simulink model "IEEE34bus_2subsystem"  (R2022b)
settings: Solver=ode4  StartTime=0.0  StopTime=inf  FixedStep=Ts  MaxStep=1e-4  RelTol=1e-4
InitFcn:
  | a=1; % Loading Factor
  | Ts=50e-6;
  | % phase to sequence conversion of RXB matrices
  | c=1*exp(sqrt(-1)*(120*pi/180));
  | T=[1 1 1;1 c*c c;1 c c*c];
  | Tinv=1/3*[1 1 1;1 c c*c;1 c*c c];
  | 
  | % Simulation data for the IEEE 34 Node Test Feeder model
  | mi2km = 1.60934;%  miles to km conversion
  | ft2km = 0.0003048; % feet to km conversion
  | ms2F = 1*1e-6/(2*pi*60);% microsiemens to Farads conversion
  | 
  | %% Configuration 300 - series reactance - ohm/mile
  | R_300 = [1.3368 0.2101 0.2130;0.2101 1.3238 0.2066;0.2130 0.2066 1.3294];
  | X_300 = [1.3343 0.5779 0.5015;0.5779 1.3569 0.4591;0.5015 0.4591 1.3471];
  | % charging susceptance - microsiemens/mile
  | B_300 = [5.3350 -1.5313 -0.9943;-1.5313 5.0979 -0.6212;-0.9943 -0.6212 4.8880];
  | 
  | R_300 = R_300/mi2km;
  | Rseq=Tinv*R_300*T;
  | R1_300=Rseq(2,2);R0_300=Rseq(1,1);
  | 
  | L_300 = (X_300/(2*pi*60))/mi2km;
  | Lseq=Tinv*L_300*T;
  | L1_300=Lseq(2,2);L0_300=Lseq(1,1);
  | 
  | C_300 =(B_300*ms2F)/mi2km;
  | Cseq=Tinv*C_300*T;
  | C1_300=Cseq(2,2);C0_300=Cseq(1,1);
  | 
  | %% Configuration 301 - series reactance - ohm/mile
  | R_301 = [1.9300 0.2327 0.2359;0.2327 1.9157 0.2288;0.2359 0.2288 1.9219];
  | X_301 = [1.4115 0.6442 0.5691;0.6442 1.4281 0.5238;0.5691 0.5238 1.4209];
  | % charging susceptance - microsiemens/mile
  | B_301 = [5.1207 -1.4364 -0.9402;-1.4364 4.9055 -0.5951;-0.9402 -0.5951 4.7154];
  | 
  | R_301 = R_301/mi2km;
  | Rseq=Tinv*R_301*T;
  | R1_301=Rseq(2,2);R0_301=Rseq(1,1);
  | 
  | L_301 = (X_301/(2*pi*60))/mi2km;
  | Lseq=Tinv*L_301*T;
  | L1_301=Lseq(2,2);L0_301=Lseq(1,1);
  | 
  | C_301 =(B_301*ms2F)/mi2km;
  | Cseq=Tinv*C_301*T;
  | C1_301=Cseq(2,2);C0_301=Cseq(1,1);
  | 
  | %% Configuration 302 - series reactance - ohm/mile
  | R_302 = [2.7995 0 0;0 0 0;0 0 0];
  | X_302 = [1.4855 0 0;0 0 0;0 0 0];
  | % charging susceptance - microsiemens/mile
  | B_302 = [4.2251 0 0;0 0 0;0 0 0];
  | 
  | R_302 = R_302/mi2km;
  | Rseq=Tinv*R_302*T;
  | R1_302=Rseq(2,2);R0_302=Rseq(1,1);
  | 
  | L_302 = (X_302/(2*pi*60))/mi2km;
  | Lseq=Tinv*L_302*T;
  | ... (+41 lines)
undefined symbols (not defined in the file): find_system, I, Left, MOV_segment19, MOV_segment9, powergui, Right, type, V, X, xn_g1
libraries: spsSeriesRLCBranchLib x75, spsGroundLib x70, spsThreePhaseVIMeasurementLib x37, spsVoltageMeasurementLib x36, spsThreePhaseSeriesRLCLoadLib x32, spsThreePhasePISectionLineLib x24, spsDCVoltageSourceLib x24, ssn_lib x16, spsSeriesRLCLoadLib x14, spsACCurrentSourceLib x12, spsOnDelayLib x12, spsPiSectionLineLib x8
(part 3 of 8)

== system IEEE34bus_2subsystem/SS_34p1/838 ==
  1 : spsThreePhaseVIMeasurementLib/Three-Phase V-I Measurement  VoltageMeasurement=phase-to-ground  SetLabelV=on  LabelV=V838  Vpu=off  VpuLL=off  CurrentMeasurement=no  SetLabelI=on  LabelI=I862  Ipu=off  Pbase=100e6  Vbase=24900  OutputType=Complex  PhasorSimulation=off  PSBequivalent=0
  Ground{1..2,9,12} (4 alike) : spsGroundLib/Ground  LConnTagsString=a
  b : PMIOPort  Side=Left
  B : PMIOPort  Port=2  Side=Right
  connections:
  1/LConn2 -- B/RConn1
  Ground12/LConn1 -- 1/LConn1
  b/RConn1 -- 1/RConn2
  Ground9/LConn1 -- 1/RConn1
  Ground2/LConn1 -- 1/LConn3
  Ground1/LConn1 -- 1/RConn3

== system IEEE34bus_2subsystem/powergui/EquivalentModel1 ==
  Sources : Subsystem
  State-Space : S-Function  FunctionName=ssn_sfun_v1  Parameters=1,0  SFunctionDeploymentMode=off  EnableBusSupport=off  SFcnStateName=MOV_segment9,MOV_segment9,MOV_segment9,MOV_segment9,MOV_segment9,MOV_segment9,MOV_segment9,MOV_segment9,MOV_segment9,MOV_segment9
      settings: SFcnIsStateOwnerBlock=on
  Yout : Subsystem
  wires:
  State-Space/1 -> Yout/1(v,i)
  Sources/1(u) -> State-Space/1

== system IEEE34bus_2subsystem/powergui/EquivalentModel2 ==
  Sources : Subsystem
  State-Space : S-Function  FunctionName=ssn_sfun_v1  Parameters=2,0  SFunctionDeploymentMode=off  EnableBusSupport=off  SFcnStateName=MOV_segment9,MOV_segment9,MOV_segment9,MOV_segment9,MOV_segment9,MOV_segment9,MOV_segment9,MOV_segment9,MOV_segment9,MOV_segment9
      settings: SFcnIsStateOwnerBlock=on
  Yout : Subsystem
  wires:
  State-Space/1 -> Yout/1(v,i)
  Sources/1(u) -> State-Space/1

== system IEEE34bus_2subsystem/powergui/EquivalentModel3 ==
  Sources : Subsystem
  State-Space : S-Function  FunctionName=ssn_sfun_v1  Parameters=3,0  SFunctionDeploymentMode=off  EnableBusSupport=off  SFcnStateName=MOV_segment9,MOV_segment9,MOV_segment9,MOV_segment9,MOV_segment9,MOV_segment9,MOV_segment9,MOV_segment9,MOV_segment9,MOV_segment9
      settings: SFcnIsStateOwnerBlock=on
  Yout : Subsystem
  wires:
  State-Space/1 -> Yout/1(v,i)
  Sources/1(u) -> State-Space/1

== system IEEE34bus_2subsystem/powergui/EquivalentModel4 ==
  Sources : Subsystem
  State-Space : S-Function  FunctionName=ssn_sfun_v1  Parameters=4,0  SFunctionDeploymentMode=off  EnableBusSupport=off  SFcnStateName=MOV_segment9,MOV_segment9,MOV_segment9,MOV_segment9,MOV_segment9,MOV_segment9,MOV_segment9,MOV_segment9,MOV_segment9,MOV_segment9
      settings: SFcnIsStateOwnerBlock=on
  Yout : Subsystem
  wires:
  State-Space/1 -> Yout/1(v,i)
  Sources/1(u) -> State-Space/1

== system IEEE34bus_2subsystem/powergui/EquivalentModel5 ==
  Sources : Subsystem
  State-Space : S-Function  FunctionName=ssn_sfun_v1  Parameters=5,0  SFunctionDeploymentMode=off  EnableBusSupport=off  SFcnStateName=MOV_segment9,MOV_segment9,MOV_segment9,MOV_segment9,MOV_segment9,MOV_segment9,MOV_segment9,MOV_segment9,MOV_segment9,MOV_segment9
      settings: SFcnIsStateOwnerBlock=on
  Yout : Subsystem
  wires:
  State-Space/1 -> Yout/1(v,i)
  Sources/1(u) -> State-Space/1

== system IEEE34bus_2subsystem/powergui/EquivalentModel6 ==
  Sources : Subsystem
  State-Space : S-Function  FunctionName=ssn_sfun_v1  Parameters=6,0  SFunctionDeploymentMode=off  EnableBusSupport=off  SFcnStateName=MOV_segment9,MOV_segment9,MOV_segment9,MOV_segment9,MOV_segment9,MOV_segment9,MOV_segment9,MOV_segment9,MOV_segment9,MOV_segment9
      settings: SFcnIsStateOwnerBlock=on
  Yout : Subsystem
  wires:
  State-Space/1 -> Yout/1(v,i)
  Sources/1(u) -> State-Space/1

== system IEEE34bus_2subsystem/powergui/EquivalentModel7 ==
  Sources : Subsystem
  State-Space : Subsystem
  Yout : Subsystem
  wires:
  State-Space/1(Out1) -> Yout/1(v,i)
  Sources/1(u) -> State-Space/1(In1)

== system IEEE34bus_2subsystem/powergui/EquivalentModel8 ==
  Sources : Subsystem
  State-Space : S-Function  FunctionName=ssn_sfun_v1  Parameters=8,0  SFunctionDeploymentMode=off  EnableBusSupport=off  SFcnStateName=MOV_segment19,xn_g1,MOV_segment19,MOV_segment19,MOV_segment19,MOV_segment19,MOV_segment19,MOV_segment19,MOV_segment19,MOV_segment19,MOV_segment19,MOV_segment19,MOV_segment19,MOV_segment19,MOV_segment19,MOV_segment19,MOV_segment19,MOV_segment19,MOV_segment19,MOV_segment19
      settings: SFcnIsStateOwnerBlock=on
  Yout : Subsystem
  wires:
  State-Space/1 -> Yout/1(v,i)
  Sources/1(u) -> State-Space/1

== system IEEE34bus_2subsystem/SM_34p/Regulator 3/Single Phase SVR_A ==
  Line Drop Compensator : Subsystem
  Transformer with Taps : Subsystem
  Voltage Regulator Control : Subsystem
  S : PMIOPort  Tag=PMCPort  Side=Left
  L : PMIOPort  Tag=PMCPort  Port=2  Side=Right
  Tap : Outport  VectorParamsAs1DForOutWhenUnconnected=off
  tag scope: Vr1a=global
  wires:
  Transformer with Taps/2(Vsec) -> Line Drop Compensator/2(Vsec)
  Transformer with Taps/1(Isec) -> Line Drop Compensator/1(Isec)
  Voltage Regulator Control/1(N) -> Transformer with Taps/1(N)
  Voltage Regulator Control/2(Tap) -> Tap/1
  Line Drop Compensator/1(Vm) -> [Vr1a], Voltage Regulator Control/1(Vm)
  connections:
  Transformer with Taps/LConn1 -- S/RConn1
  Transformer with Taps/RConn1 -- L/RConn1

== system IEEE34bus_2subsystem/SM_34p/Regulator 3/Single Phase SVR_B ==
  Line Drop Compensator : Subsystem
  Transformer with Taps : Subsystem
  Voltage Regulator Control : Subsystem
  S : PMIOPort  Tag=PMCPort  Side=Left
  L : PMIOPort  Tag=PMCPort  Port=2  Side=Right
  Tap : Outport  VectorParamsAs1DForOutWhenUnconnected=off
  tag scope: Vr1b=global
  wires:
  Line Drop Compensator/1(Vm) -> Voltage Regulator Control/1(Vm), [Vr1b]
  Voltage Regulator Control/2(Tap) -> Tap/1
  Voltage Regulator Control/1(N) -> Transformer with Taps/1(N)
  Transformer with Taps/1(Isec) -> Line Drop Compensator/1(Isec)
  Transformer with Taps/2(Vsec) -> Line Drop Compensator/2(Vsec)
  connections:
  Transformer with Taps/RConn1 -- L/RConn1
  Transformer with Taps/LConn1 -- S/RConn1

== system IEEE34bus_2subsystem/SM_34p/Regulator 3/Single Phase SVR_C ==
  Line Drop Compensator : Subsystem
  Transformer with Taps : Subsystem
  Voltage Regulator Control : Subsystem
  S : PMIOPort  Tag=PMCPort  Side=Left
  L : PMIOPort  Tag=PMCPort  Port=2  Side=Right
  Tap : Outport  VectorParamsAs1DForOutWhenUnconnected=off
  tag scope: Vr1c=global
  wires:
  Transformer with Taps/2(Vsec) -> Line Drop Compensator/2(Vsec)
  Transformer with Taps/1(Isec) -> Line Drop Compensator/1(Isec)
  Voltage Regulator Control/1(N) -> Transformer with Taps/1(N)
  Voltage Regulator Control/2(Tap) -> Tap/1
  Line Drop Compensator/1(Vm) -> [Vr1c], Voltage Regulator Control/1(Vm)
  connections:
  Transformer with Taps/LConn1 -- S/RConn1
  Transformer with Taps/RConn1 -- L/RConn1

== system IEEE34bus_2subsystem/SM_34p/Regulator 4/Single Phase SVR_A ==
  Line Drop Compensator : Subsystem
  Transformer with Taps : Subsystem
  Voltage Regulator Control : Subsystem
  S : PMIOPort  Tag=PMCPort  Side=Left
  L : PMIOPort  Tag=PMCPort  Port=2  Side=Right
  Tap : Outport  VectorParamsAs1DForOutWhenUnconnected=off
  tag scope: Vr2a=global
  wires:
  Line Drop Compensator/1(Vm) -> Voltage Regulator Control/1(Vm), [Vr2a]
  Voltage Regulator Control/2(Tap) -> Tap/1
  Voltage Regulator Control/1(N) -> Transformer with Taps/1(N)
  Transformer with Taps/1(Isec) -> Line Drop Compensator/1(Isec)
  Transformer with Taps/2(Vsec) -> Line Drop Compensator/2(Vsec)
  connections:
  Transformer with Taps/RConn1 -- L/RConn1
  Transformer with Taps/LConn1 -- S/RConn1

== system IEEE34bus_2subsystem/SM_34p/Regulator 4/Single Phase SVR_B ==
  Line Drop Compensator : Subsystem
  Transformer with Taps : Subsystem
  Voltage Regulator Control : Subsystem
  S : PMIOPort  Tag=PMCPort  Side=Left
  L : PMIOPort  Tag=PMCPort  Port=2  Side=Right
  Tap : Outport  VectorParamsAs1DForOutWhenUnconnected=off
  tag scope: Vr2b=global
  wires:
  Transformer with Taps/2(Vsec) -> Line Drop Compensator/2(Vsec)
  Transformer with Taps/1(Isec) -> Line Drop Compensator/1(Isec)
  Voltage Regulator Control/1(N) -> Transformer with Taps/1(N)
  Voltage Regulator Control/2(Tap) -> Tap/1
  Line Drop Compensator/1(Vm) -> [Vr2b], Voltage Regulator Control/1(Vm)
  connections:
  Transformer with Taps/LConn1 -- S/RConn1
  Transformer with Taps/RConn1 -- L/RConn1

== system IEEE34bus_2subsystem/SM_34p/Regulator 4/Single Phase SVR_C ==
  Line Drop Compensator : Subsystem
  Transformer with Taps : Subsystem
  Voltage Regulator Control : Subsystem
  S : PMIOPort  Tag=PMCPort  Side=Left
  L : PMIOPort  Tag=PMCPort  Port=2  Side=Right
  Tap : Outport  VectorParamsAs1DForOutWhenUnconnected=off
  tag scope: Vr2c=global
  wires:
  Line Drop Compensator/1(Vm) -> Voltage Regulator Control/1(Vm), [Vr2c]
  Voltage Regulator Control/2(Tap) -> Tap/1
  Voltage Regulator Control/1(N) -> Transformer with Taps/1(N)
  Transformer with Taps/1(Isec) -> Line Drop Compensator/1(Isec)
  Transformer with Taps/2(Vsec) -> Line Drop Compensator/2(Vsec)
  connections:
  Transformer with Taps/RConn1 -- L/RConn1
  Transformer with Taps/LConn1 -- S/RConn1

== system IEEE34bus_2subsystem/powergui/EquivalentModel1/Sources ==
  Mux : Mux  Inputs=[1 1]
  u : Outport  VectorParamsAs1DForOutWhenUnconnected=off
  wires:
  Mux/1 -> u/1
  [T91_7975_12543828221255] -> Mux/1
  [T91_7962_12463308468462] -> Mux/2

== system IEEE34bus_2subsystem/powergui/EquivalentModel1/Yout ==
  v,i : Inport
  Demux : Demux  Outputs=1
  tag scope: T94_8507_15463232269065=global
  wires:
  v,i/1 -> Demux/1
  Demux/1 -> [T94_8507_15463232269065]

== system IEEE34bus_2subsystem/powergui/EquivalentModel2/Sources ==
  Mux : Mux  Inputs=[1 1]
  u : Outport  VectorParamsAs1DForOutWhenUnconnected=off
  wires:
  Mux/1 -> u/1
  [T91_7976_12543360980049] -> Mux/1
  [T91_7963_12462866570525] -> Mux/2

== system IEEE34bus_2subsystem/powergui/EquivalentModel2/Yout ==
  v,i : Inport
  Demux : Demux  Outputs=1
  tag scope: T94_8508_15461981939973=global
  wires:
  v,i/1 -> Demux/1
  Demux/1 -> [T94_8508_15461981939973]

== system IEEE34bus_2subsystem/powergui/EquivalentModel3/Sources ==
  Mux : Mux  Inputs=[1 1]
  u : Outport  VectorParamsAs1DForOutWhenUnconnected=off
  wires:
  Mux/1 -> u/1
  [T91_7977_12543017695106] -> Mux/1
  [T91_7964_12462548628852] -> Mux/2

== system IEEE34bus_2subsystem/powergui/EquivalentModel3/Yout ==
  v,i : Inport
  Demux : Demux  Outputs=1
  tag scope: T94_8509_15460851611092=global
  wires:
  v,i/1 -> Demux/1
  Demux/1 -> [T94_8509_15460851611092]

== system IEEE34bus_2subsystem/powergui/EquivalentModel4/Sources ==
  Mux : Mux  Inputs=[1 1]
  u : Outport  VectorParamsAs1DForOutWhenUnconnected=off
  wires:
  Mux/1 -> u/1
  [T91_7976_12540912541255] -> Mux/1
  [T91_7963_12460409796462] -> Mux/2

== system IEEE34bus_2subsystem/powergui/EquivalentModel4/Yout ==
  v,i : Inport
  Demux : Demux  Outputs=1
  tag scope: T94_8508_15459874989120=global
  wires:
  v,i/1 -> Demux/1
  Demux/1 -> [T94_8508_15459874989120]

== system IEEE34bus_2subsystem/powergui/EquivalentModel5/Sources ==
  Mux : Mux  Inputs=[1 1]
  u : Outport  VectorParamsAs1DForOutWhenUnconnected=off
  wires:
  Mux/1 -> u/1
  [T91_7977_12540444375741] -> Mux/1
  [T91_7964_12459966974217] -> Mux/2

== system IEEE34bus_2subsystem/powergui/EquivalentModel5/Yout ==
  v,i : Inport
  Demux : Demux  Outputs=1
  tag scope: T94_8509_15458623794084=global
  wires:
  v,i/1 -> Demux/1
  Demux/1 -> [T94_8509_15458623794084]

== system IEEE34bus_2subsystem/powergui/EquivalentModel6/Sources ==
  Mux : Mux  Inputs=[1 1]
  u : Outport  VectorParamsAs1DForOutWhenUnconnected=off
  wires:
  Mux/1 -> u/1
  [T91_7978_12540100166491] -> Mux/1
  [T91_7965_12459648108237] -> Mux/2

== system IEEE34bus_2subsystem/powergui/EquivalentModel6/Yout ==
  v,i : Inport
  Demux : Demux  Outputs=1
  tag scope: T94_8510_15457492599260=global
  wires:
  v,i/1 -> Demux/1
  Demux/1 -> [T94_8510_15457492599260]

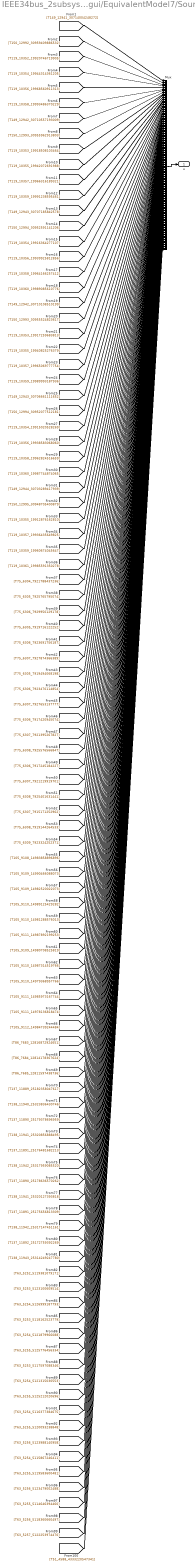
== system IEEE34bus_2subsystem/powergui/EquivalentModel7/Sources ==
  Mux : Mux  Inputs=[1 1 1 1 1 1 1 1 1 1 1 1 1 1 1 1 1 1 1 1 1 1 1 1 1 1 1 1 1 1 1 1 1 1 1 1 1 1 1 1 1 1 1 1 1 1 1 1 1 1 1 1 1 1 1 1 1 1 1 1 1 1 1 1 1 1 1 1 1 1 1 1 1 1 1 1 1 1 1 1 1 1 1 1 1 1 1 1 1 1 1 1 1 1 1 1 1 1 1 3]
  u : Outport  VectorParamsAs1DForOutWhenUnconnected=off
  wires:
  Mux/1 -> u/1
  [T149_12941_30714004248272] -> Mux/1
  [T150_12992_30959409886532] -> Mux/2
  [T119_10352_19920746719905] -> Mux/3
  [T119_10354_19944314361205] -> Mux/4
  [T119_10356_19968560911313] -> Mux/5
  [T119_10358_19993486370229] -> Mux/6
  [T149_12942_30710557193009] -> Mux/7
  [T150_12993_30955962913803] -> Mux/8
  [T119_10353_19918508103464] -> Mux/9
  [T119_10355_19942072691988] -> Mux/10
  [T119_10357_19966316189321] -> Mux/11
  [T119_10359_19991238595461] -> Mux/12
  [T149_12943_30707185842578] -> Mux/13
  [T150_12994_30952591141206] -> Mux/14
  [T119_10354_19916364277107] -> Mux/15
  [T119_10356_19939925812856] -> Mux/16
  [T119_10358_19964166257412] -> Mux/17
  [T119_10360_19989085610776] -> Mux/18
  [T149_12942_30710108510199] -> Mux/19
  [T150_12993_30955524823617] -> Mux/20
  [T119_10353_19917259683813] -> Mux/21
  [T119_10355_19940825276379] -> Mux/22
  [T119_10357_19965069777754] -> Mux/23
  [T119_10359_19989993187936] -> Mux/24
  [T149_12943_30706661111652] -> Mux/25
  [T150_12994_30952077512181] -> Mux/26
  [T119_10354_19915020528269] -> Mux/27
  [T119_10356_19938583068060] -> Mux/28
  [T119_10358_19962824516659] -> Mux/29
  [T119_10360_19987744874065] -> Mux/30
  [T149_12944_30703289417939] -> Mux/31
  [T150_12995_30948705400879] -> Mux/32
  [T119_10355_19912876162810] -> Mux/33
  [T119_10357_19936435649825] -> Mux/34
  [T119_10359_19960674045647] -> Mux/35
  [T119_10361_19985591350278] -> Mux/36
  [T75_6304_7921788437236] -> Mux/37
  [T75_6305_7925765795074] -> Mux/38
  [T75_6306_7929950129178] -> Mux/39
  [T75_6305_7919716122252] -> Mux/40
  [T75_6306_7923691756187] -> Mux/41
  [T75_6307_7927874366389] -> Mux/42
  [T75_6305_7919494068198] -> Mux/43
  [T75_6306_7923470114854] -> Mux/44
  [T75_6307_7927653137777] -> Mux/45
  [T75_6306_7917420945074] -> Mux/46
  [T75_6307_7921395267827] -> Mux/47
  [T75_6308_7925576566847] -> Mux/48
  [T75_6306_7917245184227] -> Mux/49
  [T75_6307_7921219919701] -> Mux/50
  [T75_6308_7925401631441] -> Mux/51
  [T75_6307_7915171252962] -> Mux/52
  [T75_6308_7919144264533] -> Mux/53
  [T75_6309_7923324252371] -> Mux/54
  [T105_9108_14983858896896] -> Mux/55
  [T105_9109_14990466088073] -> Mux/56
  [T105_9109_14982520022073] -> Mux/57
  [T105_9110_14989125429282] -> Mux/58
  [T105_9110_14981288576013] -> Mux/59
  [T105_9111_14987892199253] -> Mux/60
  [T105_9109_14980708525819] -> Mux/61
  [T105_9110_14987314519766] -> Mux/62
  [T105_9110_14979368957766] -> Mux/63
  [T105_9111_14985973167744] -> Mux/64
  [T105_9111_14978136818474] -> Mux/65
  [T105_9112_14984739244484] -> Mux/66
  [T86_7683_12816872924651] -> Mux/67
  [T86_7684_12814178367624] -> Mux/68
  [T86_7685_12811597438736] -> Mux/69
  [T137_11889_25182358047617] -> Mux/70
  [T138_11940_25323836430746] -> Mux/71
  [T137_11890_25179378696959] -> Mux/72
  [T138_11941_25320856888495] -> Mux/73
  [T137_11891_25176481682213] -> Mux/74
  [T138_11942_25317959085520] -> Mux/75
  [T137_11890_25178636570262] -> Mux/76
  [T138_11941_25320127393818] -> Mux/77
  [T137_11891_25175656813309] -> Mux/78
  [T138_11942_25317147451161] -> Mux/79
  [T137_11892_25172759392269] -> Mux/80
  [T138_11943_25314249247780] -> Mux/81
  [T63_5252_5119381079171] -> Mux/82
  [T63_5253_5123100609514] -> Mux/83
  [T63_5254_5126999187793] -> Mux/84
  [T63_5253_5118162523779] -> Mux/85
  [T63_5254_5121879966088] -> Mux/86
  [T63_5255_5125776456334] -> Mux/87
  [T63_5253_5117597088346] -> Mux/88
  [T63_5254_5121315030553] -> Mux/89
  [T63_5255_5125212020696] -> Mux/90
  [T63_5254_5116377384675] -> Mux/91
  [T63_5255_5120093238848] -> Mux/92
  [T63_5256_5123988140958] -> Mux/93
  [T63_5254_5115867246411] -> Mux/94
  [T63_5255_5119583600481] -> Mux/95
  [T63_5256_5123479002488] -> Mux/96
  [T63_5255_5114646394460] -> Mux/97
  [T63_5256_5118360660497] -> Mux/98
  [T63_5257_5122253974470] -> Mux/99
  [T51_4588_4333220547341] -> Mux/100

== system IEEE34bus_2subsystem/powergui/EquivalentModel7/State-Space ==
  In1 : Inport
  ssn_sfun_sw1 : S-Function  FunctionName=ssn_sfun_v1  Parameters=7,0  SFunctionDeploymentMode=off  EnableBusSupport=off  SFcnStateName=MOV_segment119,xn_g1,xn_g2,xn_g3,xn_g4,xn_g5,xn_g6,xn_g7,xn_g8,xn_g9,MOV_segment119,xn_g11,MOV_segment119,MOV_segment119,MOV_segment119,MOV_segment119,MOV_segment119,MOV_segment119,MOV_segment119,MOV_segment119,MOV_segment119,MOV_segment119,MOV_segment119,MOV_segment119,MOV_segment119,MOV_segment119,MOV_segment119,MOV_segment119,MOV_segment119,MOV_segment119,MOV_segment119,MOV_segment119,MOV_segment119,MOV_segment119,MOV_segment119,MOV_segment119,MOV_segment119,MOV_segment119,MOV_segment119,MOV_segment119,MOV_segment119,MOV_segment119,MOV_segment119,MOV_segment119,MOV_segment119,MOV_segment119,MOV_segment119,MOV_segment119,MOV_segment119,MOV_segment119,MOV_segment119,MOV_segment119,MOV_segment119,MOV_segment119,MOV_segment119,MOV_segment119,MOV_segment119,MOV_segment119,MOV_segment119,MOV_segment119,MOV_segment119,MOV_segment119,MOV_segment119,MOV_segment119,MOV_segment119,MOV_segment119,MOV_segment119,MOV_segment119,MOV_segment119,MOV_segment119,MOV_segment119,MOV_segment119,MOV_segment119,MOV_segment119,MOV_segment119,MOV_segment119,MOV_segment119,MOV_segment119,MOV_segment119,MOV_segment119,MOV_segment119,MOV_segment119,MOV_segment119,MOV_segment119,MOV_segment119,MOV_segment119,MOV_segment119,MOV_segment119,MOV_segment119,MOV_segment119,MOV_segment119,MOV_segment119,MOV_segment119,MOV_segment119,MOV_segment119,MOV_segment119,MOV_segment119,MOV_segment119,MOV_segment119,MOV_segment119,MOV_segment119,MOV_segment119,MOV_segment119,MOV_segment119,MOV_segment119,MOV_segment119,MOV_segment119,MOV_segment119,MOV_segment119,MOV_segment119,MOV_segment119,MOV_segment119,MOV_segment119,MOV_segment119,MOV_segment119,MOV_segment119,MOV_segment119,MOV_segment119,MOV_segment119,MOV_segment119
      settings: SFcnIsStateOwnerBlock=on
  Out1 : Outport  VectorParamsAs1DForOutWhenUnconnected=off
  tag scope: ssn_ext_sys_from_V_217x8a73x287908e35664=global, ssn_ext_sys_from_V_21cxb72ex3f0a0e37a867=global, ssn_ext_sys_from_V_687x9d5fx6fb80ff9f5a3=global, ssn_ext_sys_from_V_ce4x9218xa137594c517a=global, ssn_ext_sys_from_V_e41xb614x261f7399655c=global, ssn_ext_sys_from_V_e6axb282xa835046f3cfd=global
  wires:
  In1/1 -> ssn_sfun_sw1/1
  ssn_sfun_sw1/1 -> Out1/1
  [ssn_ext_sys_goto_Hist_ce4x9218xa137594c517a] -> ssn_sfun_sw1/2
  [ssn_ext_sys_goto_Y_ce4x9218xa137594c517a] -> ssn_sfun_sw1/3
  ssn_sfun_sw1/2 -> [ssn_ext_sys_from_V_ce4x9218xa137594c517a]
  [ssn_ext_sys_goto_Hist_687x9d5fx6fb80ff9f5a3] -> ssn_sfun_sw1/4
  [ssn_ext_sys_goto_Y_687x9d5fx6fb80ff9f5a3] -> ssn_sfun_sw1/5
  ssn_sfun_sw1/3 -> [ssn_ext_sys_from_V_687x9d5fx6fb80ff9f5a3]
  [ssn_ext_sys_goto_Hist_e41xb614x261f7399655c] -> ssn_sfun_sw1/6
  [ssn_ext_sys_goto_Y_e41xb614x261f7399655c] -> ssn_sfun_sw1/7
  ssn_sfun_sw1/4 -> [ssn_ext_sys_from_V_e41xb614x261f7399655c]
  [ssn_ext_sys_goto_Hist_217x8a73x287908e35664] -> ssn_sfun_sw1/8
  [ssn_ext_sys_goto_Y_217x8a73x287908e35664] -> ssn_sfun_sw1/9
  ssn_sfun_sw1/5 -> [ssn_ext_sys_from_V_217x8a73x287908e35664]
  [ssn_ext_sys_goto_Hist_21cxb72ex3f0a0e37a867] -> ssn_sfun_sw1/10
  [ssn_ext_sys_goto_Y_21cxb72ex3f0a0e37a867] -> ssn_sfun_sw1/11
  ssn_sfun_sw1/6 -> [ssn_ext_sys_from_V_21cxb72ex3f0a0e37a867]
  [ssn_ext_sys_goto_Hist_e6axb282xa835046f3cfd] -> ssn_sfun_sw1/12
  [ssn_ext_sys_goto_Y_e6axb282xa835046f3cfd] -> ssn_sfun_sw1/13
  ssn_sfun_sw1/7 -> [ssn_ext_sys_from_V_e6axb282xa835046f3cfd]

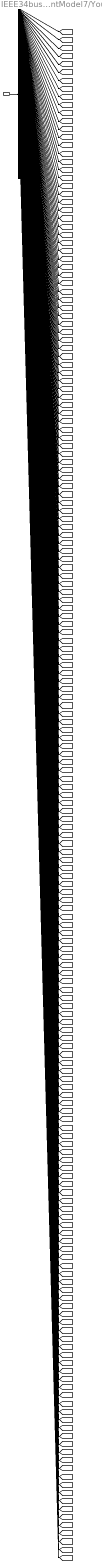
== system IEEE34bus_2subsystem/powergui/EquivalentModel7/Yout ==
  v,i : Inport
  Demux : Demux  Outputs=[1 1 1 1 1 1 1 1 1 1 1 1 1 1 1 1 1 1 1 1 1 1 1 1 1 1 1 1 1 1 1 1 1 1 1 1 1 1 1 1 1 1 1 1 1 1 1 1 1 1 1 1 1 1 1 1 1 1 1 1 1 1 1 1 1 1 1 1 1 1 1 1 1 1 1 1 1 1 1 1 1 1 1 1 1 1 1 1 1 1 1 1 1 1 1 1 1 1 1 1 1 1 1 1 1 1 1 1 1 1 1 1 1 1 1 1 1 1 1 1 1 1 1 1 1 1 1 1 1 1 1 1 1 1 1 1 1 1 1 1 1 1 1 1 1 1 1 1 1 1 1 1 1 1 1 1 1 1 1 1 1 1 1 1 1 1 1 1 1 1 1 1 1 1 1 1 1 1 1 1 1 1 1 1 1 1 1 1 1]
  tag scope: T110_9614_17346347292190=global, T110_9615_17342993552607=global, T110_9615_17344551470800=global, T110_9615_17352545003990=global, T110_9616_17341197099851=global, T110_9616_17342858195046=global, T110_9616_17349190141231=global, T110_9616_17350747508978=global, T110_9616_17359067242335=global, T110_9617_17339503192731=global, T110_9617_17347392014853=global, T110_9617_17349052559603=global, T110_9617_17355711256400=global, T110_9617_17357268073702=global, T110_9617_17365914007226=global, T110_9618_17345696434112=global, T110_9618_17353911456401=global, T110_9618_17355571450706=global, T110_9618_17362556898115=global, T110_9618_17364113164972=global, T110_9619_17352214202038=global, T110_9619_17360755424495=global, T110_9619_17362414868354=global, T110_9620_17359056496510=global, T142_12395_28279007178150=global, T142_12396_28275147940751=global, T142_12396_28275731566483=global, T142_12397_28271871950996=global, T142_12397_28272535391577=global, T142_12398_28268675398002=global, T143_12446_28477128809614=global, T143_12447_28473281648995=global, T143_12447_28473853764668=global, T143_12448_28470006231249=global, T143_12448_28470657600980=global, T143_12449_28466809694761=global, T49_4104_3617955902908=global, T49_4105_3619679371871=global, T49_4106_3615518113793=global, T49_4106_3621517493895=global, T49_4107_3614202962083=global, T49_4107_3617237977313=global, T49_4108_3615921081471=global, T49_4108_3619072493895=global, T49_4109_3612023764804=global, T49_4109_3617753853920=global, T49_4110_3611426209031=global, T49_4110_3613738278750=global, T49_4111_3613138861667=global, T49_4111_3615567445757=global, T49_4112_3609772093384=global, T49_4112_3614966167364=global, T49_4113_3607363929396=global, T49_4113_3608343918750=global, T49_4113_3611481140578=global, T49_4114_3607187124252=global, T49_4114_3609071466811=global, T49_4114_3610051690519=global, T49_4114_3613304840833=global, T49_4115_3608892683180=global, T49_4115_3610893657287=global, T49_4115_3611874115349=global, T49_4116_3610712895170=global, T49_4116_3650335588622=global, T49_4117_3603768147083=global, T49_4117_3652031800442=global, T49_4118_3605468473614=global, T49_4118_3647856656650=global, T49_4118_3653842665323=global, T49_4119_3607283453206=global, T49_4119_3646521602083=global, T49_4119_3646521713495=global, T49_4119_3649549263027=global, T49_4120_3600899341752=global, T49_4120_3648212464328=global, T49_4120_3648212692917=global, T49_4120_3651356522466=global, T49_4121_3602594435884=global, T49_4121_3644034883563=global, T49_4121_3644284781097=global, T49_4121_3644301261947=global, T49_4121_3650017979634=global, T49_4121_3650018325400=global, T49_4122_3604404183078=global, T49_4122_3643682466173=global, T49_4122_3645722257543=global, T49_4122_3645972272253=global, T49_4122_3645988518750=global, T49_4123_3645367861667=global, T49_4123_3647524284583=global, T49_4123_3647774416471=global, T49_4123_3647790428614=global, T49_4124_3641987207670=global, T49_4124_3647167910221=global, T49_4125_3639561815111=global, T49_4125_3640544478750=global, T49_4125_3643668997721=global, T49_4126_3639362432823=global, T49_4126_3641242095383=global, T49_4126_3642224993376=global, T49_4126_3645465440833=global, T49_4127_3641040734609=global, T49_4127_3643037028716=global, T49_4127_3644020161063=global, T49_4128_3642833689456=global, T49_4129_3635883747083=global, T49_4130_3637556816471=global, T49_4131_3639344538920=global, T49_4132_3632955233180=global, T49_4133_3634623070170=global, T49_4134_3636405560221=global, T50_4120_3836783074433=global, T50_4121_3836145463710=global, T50_4121_3838704166322=global, T50_4122_3838064724914=global, T50_4122_3840743197812=global, T50_4123_3840101925718=global, T50_4132_3871950385127=global, T50_4133_3870752337637=global, T50_4133_3871291858061=global, T50_4133_3873843976837=global, T50_4134_3872644329159=global, T50_4134_3873183619086=global, T50_4134_3875855508147=global, T50_4135_3874654260282=global, T50_4135_3875193319710=global, T50_4214_3757914253882=global, T50_4215_3756626744082=global, T50_4215_3759664471429=global, T50_4216_3758375130943=global, T50_4216_3761532628576=global, T50_4217_3760241457404=global, T50_4219_3761739255118=global, T50_4220_3763481241229=global, T50_4221_3765341166939=global, T51_4213_3913888470431=global, T51_4214_3912588766596=global, T51_4214_3915859784784=global, T51_4215_3914558393325=global, T51_4215_3917952328941=global, T51_4216_3910040236400=global, T51_4216_3916649249859=global, T51_4217_3912006374502=global, T51_4218_3914093742408=global, T51_4220_3905696117184=global, T51_4221_3905209944941=global, T51_4221_3907655278031=global, T51_4222_3903111774784=global, T51_4222_3907167304784=global, T51_4222_3909735668682=global, T51_4223_3902127549208=global, T51_4223_3905067673765=global, T51_4223_3909245894431=global, T51_4224_3904081647184=global, T51_4224_3907144802549=global, T51_4225_3906156974965=global, T65_5740_7084414460096=global, T65_5741_7083683141428=global, T65_5742_7083102161529=global, T68_5758_6656026278227=global, T68_5759_6653902862658=global, T68_5759_6654277366521=global, T68_5759_6659345433055=global, T68_5760_6651829614442=global, T68_5760_6652152966497=global, T68_5760_6657220585222=global, T68_5760_6657594638251=global, T68_5760_6662848146708=global, T68_5761_6650078733826=global, T68_5761_6655145904741=global, T68_5761_6655468805961=global, T68_5761_6660721866609=global, T68_5761_6661095468804=global, T68_5762_6653393141025=global, T68_5762_6658645753863=global, T68_5762_6658968204249=global, T68_5763_6656891107048=global, T90_8139_13615949796674=global, T90_8140_13612757086921=global, T90_8140_13615113322373=global, T90_8141_13611919667542=global, T90_8141_13614402181628=global, T90_8142_13611207581718=global, T91_8175_13525563263162=global, T91_8176_13522412737624=global, T91_8176_13524746083465=global, T91_8177_13521594633619=global, T91_8177_13524052860032=global, T91_8178_13520900485878=global
  wires:
  v,i/1 -> Demux/1
  Demux/1 -> [T49_4116_3650335588622]
  Demux/2 -> [T49_4117_3652031800442]
  Demux/3 -> [T49_4118_3653842665323]
  Demux/4 -> [T49_4118_3647856656650]
  Demux/5 -> [T49_4119_3649549263027]
  Demux/6 -> [T49_4120_3651356522466]
  Demux/7 -> [T49_4122_3643682466173]
  Demux/8 -> [T49_4123_3645367861667]
  Demux/9 -> [T49_4124_3647167910221]
  Demux/10 -> [T49_4124_3641987207670]
  Demux/11 -> [T49_4125_3643668997721]
  Demux/12 -> [T49_4126_3645465440833]
  Demux/13 -> [T51_4213_3913888470431]
  Demux/14 -> [T51_4214_3915859784784]
  Demux/15 -> [T51_4215_3917952328941]
  Demux/16 -> [T49_4119_3646521602083]
  Demux/17 -> [T49_4120_3648212464328]
  Demux/18 -> [T49_4121_3650017979634]
  Demux/19 -> [T49_4121_3644301261947]
  Demux/20 -> [T49_4122_3645988518750]
  Demux/21 -> [T49_4123_3647790428614]
  Demux/22 -> [T50_4133_3871291858061]
  Demux/23 -> [T50_4134_3873183619086]
  Demux/24 -> [T50_4135_3875193319710]
  Demux/25 -> [T51_4221_3905209944941]
  Demux/26 -> [T51_4222_3907167304784]
  Demux/27 -> [T51_4223_3909245894431]
  Demux/28 -> [T51_4214_3912588766596]
  Demux/29 -> [T51_4215_3914558393325]
  Demux/30 -> [T51_4216_3916649249859]
  Demux/31 -> [T51_4216_3910040236400]
  Demux/32 -> [T51_4217_3912006374502]
  Demux/33 -> [T51_4218_3914093742408]
  Demux/34 -> [T50_4132_3871950385127]
  Demux/35 -> [T50_4133_3873843976837]
  Demux/36 -> [T50_4134_3875855508147]
  Demux/37 -> [T51_4220_3905696117184]
  Demux/38 -> [T51_4221_3907655278031]
  Demux/39 -> [T51_4222_3909735668682]
  Demux/40 -> [T49_4126_3639362432823]
  Demux/41 -> [T49_4127_3641040734609]
  Demux/42 -> [T49_4128_3642833689456]
  Demux/43 -> [T49_4119_3646521713495]
  Demux/44 -> [T49_4120_3648212692917]
  Demux/45 -> [T49_4121_3650018325400]
  Demux/46 -> [T49_4121_3644034883563]
  Demux/47 -> [T49_4122_3645722257543]
  Demux/48 -> [T49_4123_3647524284583]
  Demux/49 -> [T49_4121_3644284781097]
  Demux/50 -> [T49_4122_3645972272253]
  Demux/51 -> [T49_4123_3647774416471]
  Demux/52 -> [T50_4133_3870752337637]
  Demux/53 -> [T50_4134_3872644329159]
  Demux/54 -> [T50_4135_3874654260282]
  Demux/55 -> [T49_4125_3639561815111]
  Demux/56 -> [T49_4126_3641242095383]
  Demux/57 -> [T49_4127_3643037028716]
  Demux/58 -> [T51_4223_3902127549208]
  Demux/59 -> [T51_4224_3904081647184]
  Demux/60 -> [T51_4225_3906156974965]
  Demux/61 -> [T49_4129_3635883747083]
  Demux/62 -> [T49_4130_3637556816471]
  Demux/63 -> [T49_4131_3639344538920]
  Demux/64 -> [T51_4222_3903111774784]
  Demux/65 -> [T51_4223_3905067673765]
  Demux/66 -> [T51_4224_3907144802549]
  Demux/67 -> [T49_4132_3632955233180]
  Demux/68 -> [T49_4133_3634623070170]
  Demux/69 -> [T49_4134_3636405560221]
  Demux/70 -> [T49_4125_3640544478750]
  Demux/71 -> [T49_4126_3642224993376]
  Demux/72 -> [T49_4127_3644020161063]
  Demux/73 -> [T50_4214_3757914253882]
  Demux/74 -> [T50_4215_3759664471429]
  Demux/75 -> [T50_4216_3761532628576]
  Demux/76 -> [T50_4215_3756626744082]
  Demux/77 -> [T50_4216_3758375130943]
  Demux/78 -> [T50_4217_3760241457404]
  Demux/79 -> [T90_8139_13615949796674]
  Demux/80 -> [T142_12395_28279007178150]
  Demux/81 -> [T143_12446_28477128809614]
  Demux/82 -> [T110_9614_17346347292190]
  Demux/83 -> [T110_9615_17352545003990]
  Demux/84 -> [T110_9616_17359067242335]
  Demux/85 -> [T110_9617_17365914007226]
  Demux/86 -> [T90_8140_13615113322373]
  Demux/87 -> [T142_12396_28275731566483]
  Demux/88 -> [T143_12447_28473853764668]
  Demux/89 -> [T110_9615_17344551470800]
  Demux/90 -> [T110_9616_17350747508978]
  Demux/91 -> [T110_9617_17357268073702]
  Demux/92 -> [T110_9618_17364113164972]
  Demux/93 -> [T90_8141_13614402181628]
  Demux/94 -> [T142_12397_28272535391577]
  Demux/95 -> [T143_12448_28470657600980]
  Demux/96 -> [T110_9616_17342858195046]
  Demux/97 -> [T110_9617_17349052559603]
  Demux/98 -> [T110_9618_17355571450706]
  Demux/99 -> [T110_9619_17362414868354]
  Demux/100 -> [T90_8140_13612757086921]
  Demux/101 -> [T142_12396_28275147940751]
  Demux/102 -> [T143_12447_28473281648995]
  Demux/103 -> [T110_9615_17342993552607]
  Demux/104 -> [T110_9616_17349190141231]
  Demux/105 -> [T110_9617_17355711256400]
  Demux/106 -> [T110_9618_17362556898115]
  Demux/107 -> [T90_8141_13611919667542]
  Demux/108 -> [T142_12397_28271871950996]
  Demux/109 -> [T143_12448_28470006231249]
  Demux/110 -> [T110_9616_17341197099851]
  Demux/111 -> [T110_9617_17347392014853]
  Demux/112 -> [T110_9618_17353911456401]
  Demux/113 -> [T110_9619_17360755424495]
  Demux/114 -> [T90_8142_13611207581718]
  Demux/115 -> [T142_12398_28268675398002]
  Demux/116 -> [T143_12449_28466809694761]
  Demux/117 -> [T110_9617_17339503192731]
  Demux/118 -> [T110_9618_17345696434112]
  Demux/119 -> [T110_9619_17352214202038]
  Demux/120 -> [T110_9620_17359056496510]
  Demux/121 -> [T68_5758_6656026278227]
  Demux/122 -> [T68_5759_6659345433055]
  Demux/123 -> [T68_5760_6662848146708]
  Demux/124 -> [T68_5759_6654277366521]
  Demux/125 -> [T68_5760_6657594638251]
  Demux/126 -> [T68_5761_6661095468804]
  Demux/127 -> [T68_5759_6653902862658]
  Demux/128 -> [T68_5760_6657220585222]
  Demux/129 -> [T68_5761_6660721866609]
  Demux/130 -> [T68_5760_6652152966497]
  Demux/131 -> [T68_5761_6655468805961]
  Demux/132 -> [T68_5762_6658968204249]
  Demux/133 -> [T68_5760_6651829614442]
  Demux/134 -> [T68_5761_6655145904741]
  Demux/135 -> [T68_5762_6658645753863]
  Demux/136 -> [T68_5761_6650078733826]
  Demux/137 -> [T68_5762_6653393141025]
  Demux/138 -> [T68_5763_6656891107048]
  Demux/139 -> [T50_4219_3761739255118]
  Demux/140 -> [T50_4220_3763481241229]
  Demux/141 -> [T50_4221_3765341166939]
  Demux/142 -> [T65_5740_7084414460096]
  Demux/143 -> [T65_5741_7083683141428]
  Demux/144 -> [T65_5742_7083102161529]
  Demux/145 -> [T49_4104_3617955902908]
  Demux/146 -> [T49_4105_3619679371871]
  Demux/147 -> [T49_4106_3621517493895]
  Demux/148 -> [T49_4106_3615518113793]
  Demux/149 -> [T49_4107_3617237977313]
  Demux/150 -> [T49_4108_3619072493895]
  Demux/151 -> [T49_4110_3611426209031]
  Demux/152 -> [T49_4111_3613138861667]
  Demux/153 -> [T49_4112_3614966167364]
  Demux/154 -> [T49_4112_3609772093384]
  Demux/155 -> [T49_4113_3611481140578]
  Demux/156 -> [T49_4114_3613304840833]
  Demux/157 -> [T49_4107_3614202962083]
  Demux/158 -> [T49_4108_3615921081471]
  Demux/159 -> [T49_4109_3617753853920]
  Demux/160 -> [T49_4109_3612023764804]
  Demux/161 -> [T49_4110_3613738278750]
  Demux/162 -> [T49_4111_3615567445757]
  Demux/163 -> [T50_4121_3836145463710]
  Demux/164 -> [T50_4122_3838064724914]
  Demux/165 -> [T50_4123_3840101925718]
  Demux/166 -> [T50_4120_3836783074433]
  Demux/167 -> [T50_4121_3838704166322]
  Demux/168 -> [T50_4122_3840743197812]
  Demux/169 -> [T49_4114_3607187124252]
  Demux/170 -> [T49_4115_3608892683180]
  Demux/171 -> [T49_4116_3610712895170]
  Demux/172 -> [T49_4113_3607363929396]
  Demux/173 -> [T49_4114_3609071466811]
  Demux/174 -> [T49_4115_3610893657287]
  Demux/175 -> [T49_4117_3603768147083]
  Demux/176 -> [T49_4118_3605468473614]
  Demux/177 -> [T49_4119_3607283453206]
  Demux/178 -> [T49_4120_3600899341752]
  Demux/179 -> [T49_4121_3602594435884]
  Demux/180 -> [T49_4122_3604404183078]
  Demux/181 -> [T49_4113_3608343918750]
  Demux/182 -> [T49_4114_3610051690519]
  Demux/183 -> [T49_4115_3611874115349]
  Demux/184 -> [T91_8175_13525563263162]
  Demux/185 -> [T91_8176_13524746083465]
  Demux/186 -> [T91_8177_13524052860032]
  Demux/187 -> [T91_8176_13522412737624]
  Demux/188 -> [T91_8177_13521594633619]
  Demux/189 -> [T91_8178_13520900485878]

== system IEEE34bus_2subsystem/powergui/EquivalentModel8/Sources ==
  Mux : Mux  Inputs=[1 1 1 1 1 1 1 1 1 1 1 1 1 1 1]
  u : Outport  VectorParamsAs1DForOutWhenUnconnected=off
  wires:
  Mux/1 -> u/1
  [T76_6362_8157671371865] -> Mux/1
  [T76_6363_8161760195360] -> Mux/2
  [T76_6364_8166059344118] -> Mux/3
  [T76_6363_8155613182770] -> Mux/4
  [T76_6364_8159700262181] -> Mux/5
  [T76_6365_8163997666854] -> Mux/6
  [T86_7684_12813851395750] -> Mux/7
  [T86_7685_12811155999157] -> Mux/8
  [T86_7686_12808574230705] -> Mux/9
  [T64_5310_5295653632001] -> Mux/10
  [T64_5311_5299492212815] -> Mux/11
  [T64_5312_5303513198628] -> Mux/12
  [T64_5311_5294472482259] -> Mux/13
  [T64_5312_5298308956009] -> Mux/14
  [T64_5313_5302327834759] -> Mux/15

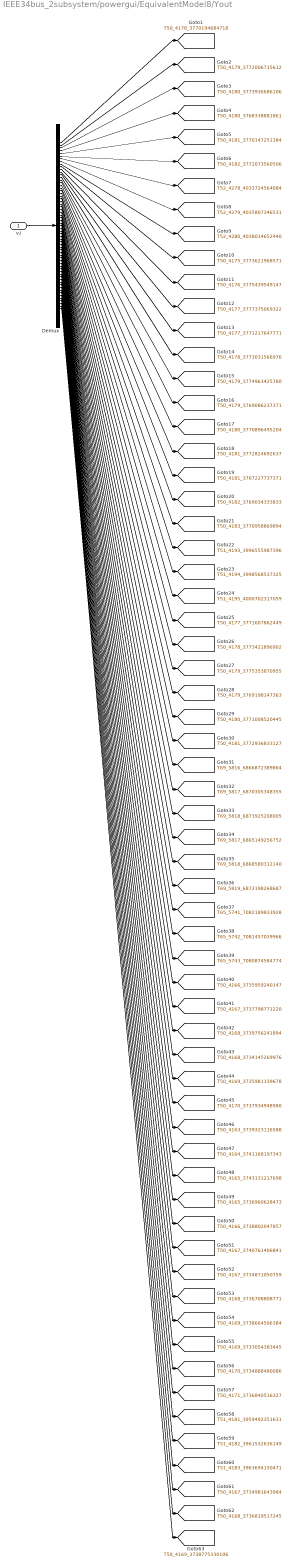
== system IEEE34bus_2subsystem/powergui/EquivalentModel8/Yout ==
  v,i : Inport
  Demux : Demux  Outputs=[1 1 1 1 1 1 1 1 1 1 1 1 1 1 1 1 1 1 1 1 1 1 1 1 1 1 1 1 1 1 1 1 1 1 1 1 1 1 1 1 1 1 1 1 1 1 1 1 1 1 1 1 1 1 1 1 1 1 1 1 1 1 1]
  tag scope: T50_4163_3739323116588=global, T50_4164_3741168197343=global, T50_4165_3736960628473=global, T50_4165_3743131217698=global, T50_4166_3735959240147=global, T50_4166_3738802047857=global, T50_4167_3734871050759=global, T50_4167_3734981643984=global, T50_4167_3737798771220=global, T50_4167_3740761406841=global, T50_4168_3734145269976=global, T50_4168_3736708808771=global, T50_4168_3736819517245=global, T50_4168_3739756241894=global, T50_4169_3733054383445=global, T50_4169_3735981139678=global, T50_4169_3738664506384=global, T50_4169_3738775330106=global, T50_4170_3734888480086=global, T50_4170_3737934948980=global, T50_4171_3736840516327=global, T50_4175_3773621968571=global, T50_4176_3775439549147=global, T50_4177_3771217647771=global, T50_4177_3771607862449=global, T50_4177_3777375069322=global, T50_4178_3770194684718=global, T50_4178_3773031566976=global, T50_4178_3773421896902=global, T50_4179_3769086237371=global, T50_4179_3769198147363=global, T50_4179_3772006715612=global, T50_4179_3774963425780=global, T50_4179_3775353870955=global, T50_4180_3768338881861=global, T50_4180_3770896495204=global, T50_4180_3771008520445=global, T50_4180_3773936686106=global, T50_4181_3767227737371=global, T50_4181_3770147251384=global, T50_4181_3772824692637=global, T50_4181_3772936833127=global, T50_4182_3769034333833=global, T50_4182_3772073560506=global, T50_4183_3770958869894=global, T51_4181_3959492351631=global, T51_4182_3961532636149=global, T51_4183_3963694150471=global, T51_4193_3996555987396=global, T51_4194_3998568537325=global, T51_4195_4000702317059=global, T52_4278_4033724564084=global, T52_4279_4035807346531=global, T52_4280_4038014652440=global, T65_5741_7082189833928=global, T65_5742_7081457039966=global, T65_5743_7080874584774=global, T69_5816_6866872389864=global, T69_5817_6865149256752=global, T69_5817_6870305348355=global, T69_5818_6868580312140=global, T69_5818_6873925208005=global, T69_5819_6872198268687=global
  wires:
  v,i/1 -> Demux/1
  Demux/1 -> [T50_4178_3770194684718]
  Demux/2 -> [T50_4179_3772006715612]
  Demux/3 -> [T50_4180_3773936686106]
  Demux/4 -> [T50_4180_3768338881861]
  Demux/5 -> [T50_4181_3770147251384]
  Demux/6 -> [T50_4182_3772073560506]
  Demux/7 -> [T52_4278_4033724564084]
  Demux/8 -> [T52_4279_4035807346531]
  Demux/9 -> [T52_4280_4038014652440]
  Demux/10 -> [T50_4175_3773621968571]
  Demux/11 -> [T50_4176_3775439549147]
  Demux/12 -> [T50_4177_3777375069322]
  Demux/13 -> [T50_4177_3771217647771]
  Demux/14 -> [T50_4178_3773031566976]
  Demux/15 -> [T50_4179_3774963425780]
  Demux/16 -> [T50_4179_3769086237371]
  Demux/17 -> [T50_4180_3770896495204]
  Demux/18 -> [T50_4181_3772824692637]
  Demux/19 -> [T50_4181_3767227737371]
  Demux/20 -> [T50_4182_3769034333833]
  Demux/21 -> [T50_4183_3770958869894]
  Demux/22 -> [T51_4193_3996555987396]
  Demux/23 -> [T51_4194_3998568537325]
  Demux/24 -> [T51_4195_4000702317059]
  Demux/25 -> [T50_4177_3771607862449]
  Demux/26 -> [T50_4178_3773421896902]
  Demux/27 -> [T50_4179_3775353870955]
  Demux/28 -> [T50_4179_3769198147363]
  Demux/29 -> [T50_4180_3771008520445]
  Demux/30 -> [T50_4181_3772936833127]
  Demux/31 -> [T69_5816_6866872389864]
  Demux/32 -> [T69_5817_6870305348355]
  Demux/33 -> [T69_5818_6873925208005]
  Demux/34 -> [T69_5817_6865149256752]
  Demux/35 -> [T69_5818_6868580312140]
  Demux/36 -> [T69_5819_6872198268687]
  Demux/37 -> [T65_5741_7082189833928]
  Demux/38 -> [T65_5742_7081457039966]
  Demux/39 -> [T65_5743_7080874584774]
  Demux/40 -> [T50_4166_3735959240147]
  Demux/41 -> [T50_4167_3737798771220]
  Demux/42 -> [T50_4168_3739756241894]
  Demux/43 -> [T50_4168_3734145269976]
  Demux/44 -> [T50_4169_3735981139678]
  Demux/45 -> [T50_4170_3737934948980]
  Demux/46 -> [T50_4163_3739323116588]
  Demux/47 -> [T50_4164_3741168197343]
  Demux/48 -> [T50_4165_3743131217698]
  Demux/49 -> [T50_4165_3736960628473]
  Demux/50 -> [T50_4166_3738802047857]
  Demux/51 -> [T50_4167_3740761406841]
  Demux/52 -> [T50_4167_3734871050759]
  Demux/53 -> [T50_4168_3736708808771]
  Demux/54 -> [T50_4169_3738664506384]
  Demux/55 -> [T50_4169_3733054383445]
  Demux/56 -> [T50_4170_3734888480086]
  Demux/57 -> [T50_4171_3736840516327]
  Demux/58 -> [T51_4181_3959492351631]
  Demux/59 -> [T51_4182_3961532636149]
  Demux/60 -> [T51_4183_3963694150471]
  Demux/61 -> [T50_4167_3734981643984]
  Demux/62 -> [T50_4168_3736819517245]
  Demux/63 -> [T50_4169_3738775330106]

== system IEEE34bus_2subsystem/SM_34p/Regulator 3/Single Phase SVR_A/Line Drop Compensator ==
  note: Vm=Vsec-Isec(Rc+jXc)
  Isec : Inport
  Vsec : Inport  Port=2
  "        " : spsLinearTransformerLib/Linear Transformer  UNITS=SI  NominalPower=[pNom fNom]  winding1=[vNom/ptRatio 1e-7 1e-8]  winding2=[vNom/ptRatio 1e-7 1e-8]  ThreeWindings=off  winding3=[3.15e+005 0.7938 0.084225]  RmLm=[1e5 1e5]  Measurements=None  DataType=on
  "CTS  " : spsControlledCurrentSourceLib/Controlled Current Source  Initialize=on  Source_Type=AC  Amplitude=0  Phase=0  Frequency=0  Measurements=None
  "PTS  " : spsControlledVoltageSourceLib/Controlled Voltage Source  Initialize=on  Source_Type=AC  Amplitude=0  Phase=0  Frequency=0  Measurements=None
  RMS : spsRMSLib/RMS  TrueRMS=on  Freq=60  RMSInit=120  Ts=0
  Raux : spsSeriesRLCBranchLib/Series RLC Branch  LConnTagsString=__new0  RConnTagsString=__new0  BranchType=R  Resistance=1e3  Inductance=1.6 / (120*pi)  SetiL0=off  InitialCurrent=0  Capacitance=1e-6  Setx0=off  InitialVoltage=0  Measurements=None
  Rc+jXc : spsSeriesRLCBranchLib/Series RLC Branch  LConnTagsString=__new0  RConnTagsString=__new0  BranchType=RL  Resistance=Rc  Inductance=Xc / (2*pi*fNom)  SetiL0=off  InitialCurrent=0  Capacitance=1e-6  Setx0=off  InitialVoltage=0  Measurements=None
  VRelay : spsVoltageMeasurementLib/Voltage Measurement  PhasorSimulation=off  OutputType=Complex  PSBequivalent=0
  Vm : Outport
  wires:
  Vsec/1 -> "PTS  "/1
  Isec/1 -> "CTS  "/1
  VRelay/1 -> RMS/1
  RMS/1 -> Vm/1
  connections:
  VRelay/LConn2 -- "PTS  "/LConn1
  "        "/LConn2 -- "CTS  "/LConn1 -- Raux/RConn1 -- Rc+jXc/RConn1
  "CTS  "/RConn1 -- "        "/LConn1 -- Rc+jXc/LConn1 -- Raux/LConn1
  "        "/RConn2 -- VRelay/LConn1
  "PTS  "/RConn1 -- "        "/RConn1
